simulink model "CACC_3_vehicles"  (R2021a)
settings: Solver=VariableStepAuto  StartTime=0.0  StopTime=120  RelTol=1e-3
values from neighbouring files (symbols this model uses):
  h = 0.9    [CACC_6_vehicles.m]    (also in CACC_6_vehicles_with_independent_FF_of_LeadVeh_Acceltn_Pstn.m; CACC_init.m)
  Kd = 1.2    [CACC_6_vehicles.m]    (also in CACC_6_vehicles_with_independent_FF_of_LeadVeh_Acceltn_Pstn.m; CACC_init.m)
  Kp = 1.5    [CACC_6_vehicles.m]    (also in CACC_6_vehicles_with_independent_FF_of_LeadVeh_Acceltn_Pstn.m; CACC_init.m)
  Lambda0 = 1    [CACC_6_vehicles.m]    (also in CACC_6_vehicles_with_independent_FF_of_LeadVeh_Acceltn_Pstn.m; CACC_init.m)
  Lambda1 = 0.5    [CACC_6_vehicles.m]    (also in CACC_6_vehicles_with_independent_FF_of_LeadVeh_Acceltn_Pstn.m; CACC_init.m)
  Lambda2 = 0.7    [CACC_6_vehicles.m]    (also in CACC_6_vehicles_with_independent_FF_of_LeadVeh_Acceltn_Pstn.m; CACC_init.m)
  Lambda3 = 0.75    [CACC_6_vehicles.m]    (also in CACC_6_vehicles_with_independent_FF_of_LeadVeh_Acceltn_Pstn.m; CACC_init.m)
  tau = 0.002    [CACC_6_vehicles.m]    (also in CACC_6_vehicles_with_independent_FF_of_LeadVeh_Acceltn_Pstn.m; CACC_init.m)
  tau0 = 0.1    [CACC_6_vehicles.m]    (also in CACC_6_vehicles_with_independent_FF_of_LeadVeh_Acceltn_Pstn.m; CACC_init.m)
  tau1 = 0.5    [CACC_6_vehicles.m]    (also in CACC_6_vehicles_with_independent_FF_of_LeadVeh_Acceltn_Pstn.m; CACC_init.m)
  tau2 = 0.7    [CACC_6_vehicles.m]    (also in CACC_6_vehicles_with_independent_FF_of_LeadVeh_Acceltn_Pstn.m; CACC_init.m)
  tau3 = 0.3    [CACC_6_vehicles.m]    (also in CACC_6_vehicles_with_independent_FF_of_LeadVeh_Acceltn_Pstn.m; CACC_init.m)
undefined symbols (not defined in the file or in its folder): sigbuilder_block
libraries: pid_lib x3
settings Model: Creator=ChOm1  LastModifiedBy=User
settings SolverCC: AlgebraicLoopSolver=TrustRegion
settings DebuggingCC: SFMachineParentedDataDiag=warning

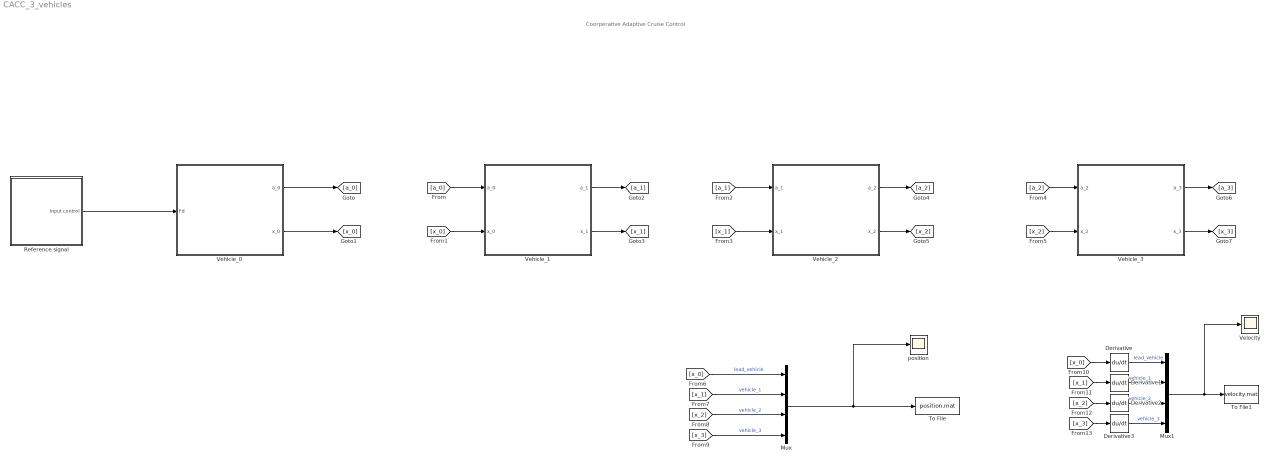
== system CACC_3_vehicles ==
  note: Coorperative Adaptive Cruise Control
  Derivative{,1..3} (4 alike) : Derivative
  Mux : Mux
  Mux1 : Mux
  Reference signal : Subsystem  Tag=STV Subsys  LoadFcn=sigbuilder_block('load');  StartFcn=sigbuilder_block('start');  StopFcn=sigbuilder_block('stop');  ClipboardFcn=sigbuilder_block('clipboard');  mask(Sigbuilder block){tuvar=[0:10]}
      mask help: Simulink:masks:SigbuilderBlock_MD
      mask init:
      | if ~strcmp(get_param(bdroot(gcbh),'SimulationStatus'),'stopped') tuvar = sigbuilder_block('maskInit'); end
      settings: CopyFcn=sigbuilder_block('copy');  DeleteFcn=sigbuilder_block('delete');  ModelCloseFcn=sigbuilder_block('modelClose');  PreSaveFcn=sigbuilder_block('preSave');  PauseFcn=sigbuilder_block('pause');  ContinueFcn=sigbuilder_block('continue');  NameChangeFcn=sigbuilder_block('namechange');  OpenFcn=sigbuilder_block('open',[259.5 231.75 543.75 273.75 ]);  CloseFcn=sigbuilder_block('close');
      mask Display: plot(0, 0, 100, 100,[2, 2, 32, 32, 2], [68, 8, 8, 68, 68],[32, 2], [38, 38], [32, 19, 2],[53, 60, 44], [32, 17, 17, 2],[16, 16, 31, 31]);txt = getActiveGroup(gcbh);text(2, 100, txt,'verticalAlignment', 'top');
  To File : ToFile  Filename=position.mat
  To File1 : ToFile  Filename=velocity.mat
  Vehicle_0 : Subsystem
  Vehicle_1 : Subsystem
  Vehicle_2 : Subsystem
  Vehicle_3 : Subsystem
  Velocity : Scope
  position : Scope
  wires:
  Reference signal/1(Input control) -> Vehicle_0/1(Fd)
  Vehicle_0/1(a_0) -> [a_0]
  Vehicle_0/2(x_0) -> [x_0]
  [a_0] -> Vehicle_1/1(a_0)
  [x_0] -> Vehicle_1/2(x_0)
  Vehicle_1/1(a_1) -> [a_1]
  [a_1] -> Vehicle_2/1(a_1)
  [x_1] -> Vehicle_2/2(x_1)
  Vehicle_2/1(a_2) -> [a_2]
  Vehicle_2/2(x_2) -> [x_2]
  [x_2] -> Vehicle_3/2(x_2)
  [a_2] -> Vehicle_3/1(a_2)
  Vehicle_3/1(a_3) -> [a_3]
  Vehicle_3/2(x_3) -> [x_3]
  Vehicle_1/2(x_1) -> [x_1]
  [x_0] -> Mux/1  "lead_vehicle"
  [x_1] -> Mux/2  "vehicle_1"
  [x_2] -> Mux/3  "vehicle_2"
  [x_3] -> Mux/4  "vehicle_3"
  Mux/1 -> position/1, To File/1
  [x_2] -> Derivative2/1
  Mux1/1 -> Velocity/1, To File1/1
  [x_0] -> Derivative/1
  Derivative/1 -> Mux1/1  "lead_vehicle"
  [x_1] -> Derivative1/1
  Derivative1/1 -> Mux1/2  "vehicle_1"
  Derivative2/1 -> Mux1/3  "vehicle_2"
  [x_3] -> Derivative3/1
  Derivative3/1 -> Mux1/4  "vehicle_3"

== system CACC_3_vehicles/Reference signal ==
  Demux : Demux  Tag=STV Demux  Outputs=1
      settings: DisplayOption=none
  FromWs : FromWorkspace  Tag=STV FromWs  VariableName=tuvar
      SigBuilderData=|
      | common.afterFinalStr = 'Extrapolate'
      | common.sampleTime = 0
      | dataSet.timeRange = [0 120]
      | dataSet.name = 'Group 1'
      | sbobj.Groups.Name = 'Group 1'
      | sbobj.Groups.Signals.Name = 'Input control'
      | sbobj.Groups.Signals.XData = [0 20.1 20.1 23.5 23.5 27.9 27.9 51.7 60.1 85.2 110.5 120]
      | sbobj.Groups.Signals.YData = [0 1.045 -1.5 -0.64 1.86 2.08 2.09 0 0 -2 0 0]
      | sbobj.Groups.TimeRange = [0 120]
  Input control : Outport  Tag=STV Outport
  wires:
  FromWs/1 -> Demux/1
  Demux/1 -> Input control/1

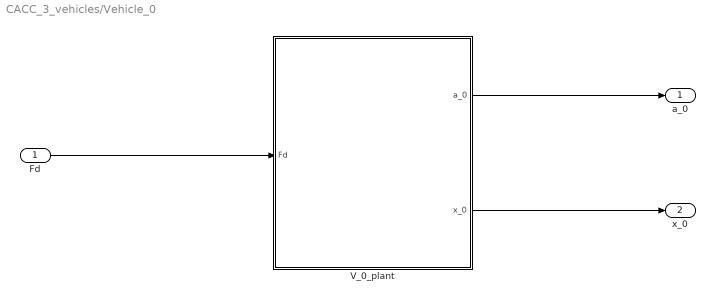
== system CACC_3_vehicles/Vehicle_0 ==
  Fd : Inport
  V_0_plant : Subsystem
  a_0 : Outport
  x_0 : Outport  Port=2
  wires:
  Fd/1 -> V_0_plant/1(Fd)
  V_0_plant/1(a_0) -> a_0/1
  V_0_plant/2(x_0) -> x_0/1

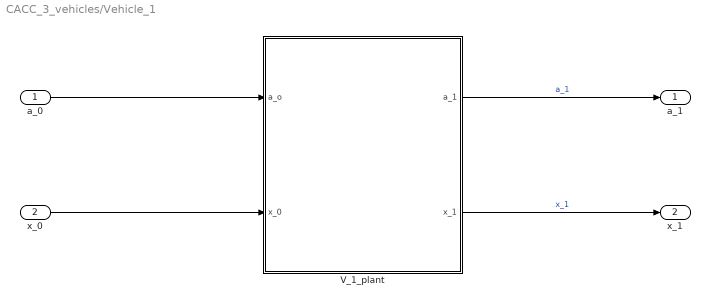
== system CACC_3_vehicles/Vehicle_1 ==
  a_0 : Inport
  x_0 : Inport  Port=2
  V_1_plant : Subsystem
  a_1 : Outport
  x_1 : Outport  Port=2
  wires:
  a_0/1 -> V_1_plant/1(a_o)
  x_0/1 -> V_1_plant/2(x_0)
  V_1_plant/1(a_1) -> a_1/1  "a_1"
  V_1_plant/2(x_1) -> x_1/1  "x_1"

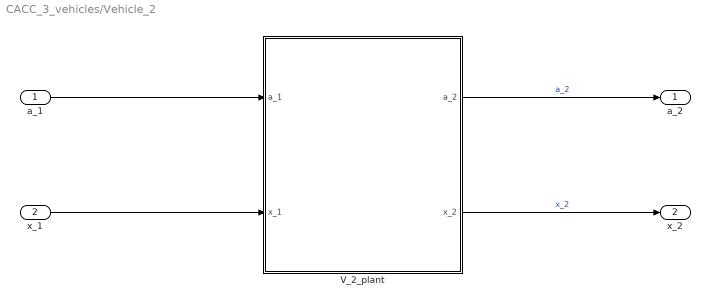
== system CACC_3_vehicles/Vehicle_2 ==
  a_1 : Inport
  x_1 : Inport  Port=2
  V_2_plant : Subsystem
  a_2 : Outport
  x_2 : Outport  Port=2
  wires:
  V_2_plant/2(x_2) -> x_2/1  "x_2"
  V_2_plant/1(a_2) -> a_2/1  "a_2"
  x_1/1 -> V_2_plant/2(x_1)
  a_1/1 -> V_2_plant/1(a_1)

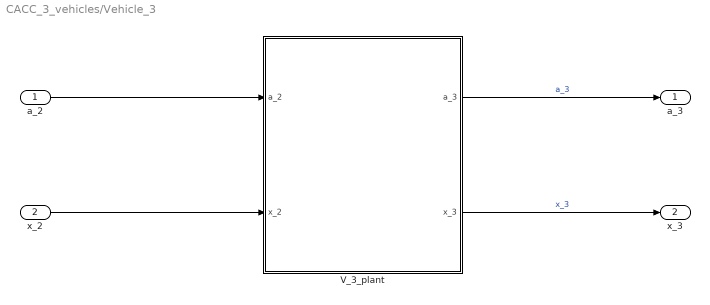
== system CACC_3_vehicles/Vehicle_3 ==
  a_2 : Inport
  x_2 : Inport  Port=2
  V_3_plant : Subsystem
  a_3 : Outport
  x_3 : Outport  Port=2
  wires:
  a_2/1 -> V_3_plant/1(a_2)
  x_2/1 -> V_3_plant/2(x_2)
  V_3_plant/1(a_3) -> a_3/1  "a_3"
  V_3_plant/2(x_3) -> x_3/1  "x_3"

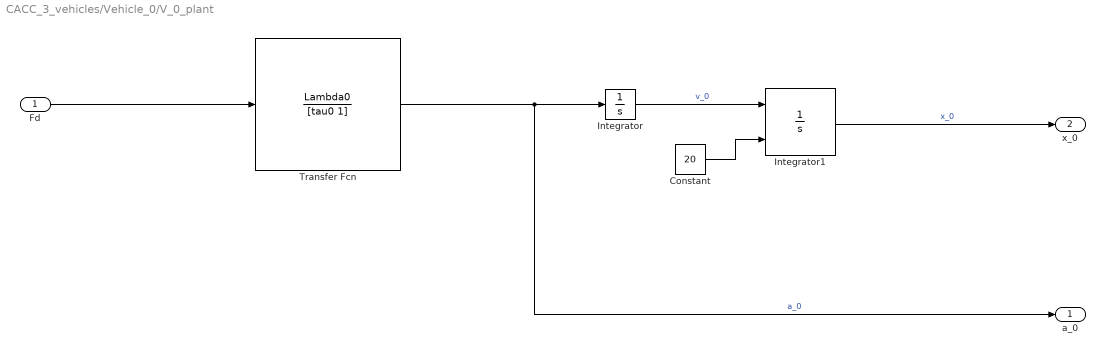
== system CACC_3_vehicles/Vehicle_0/V_0_plant ==
  Fd : Inport
  Constant : Constant  Value=20
  Integrator : Integrator
  Integrator1 : Integrator  InitialConditionSource=external
  Transfer Fcn : TransferFcn  Numerator=Lambda0  Denominator=[tau0 1]
  a_0 : Outport
  x_0 : Outport  Port=2
  wires:
  Fd/1 -> Transfer Fcn/1
  Transfer Fcn/1 -> a_0/1, Integrator/1  "a_0"
  Integrator/1 -> Integrator1/1  "v_0"
  Integrator1/1 -> x_0/1  "x_0"
  Constant/1 -> Integrator1/2

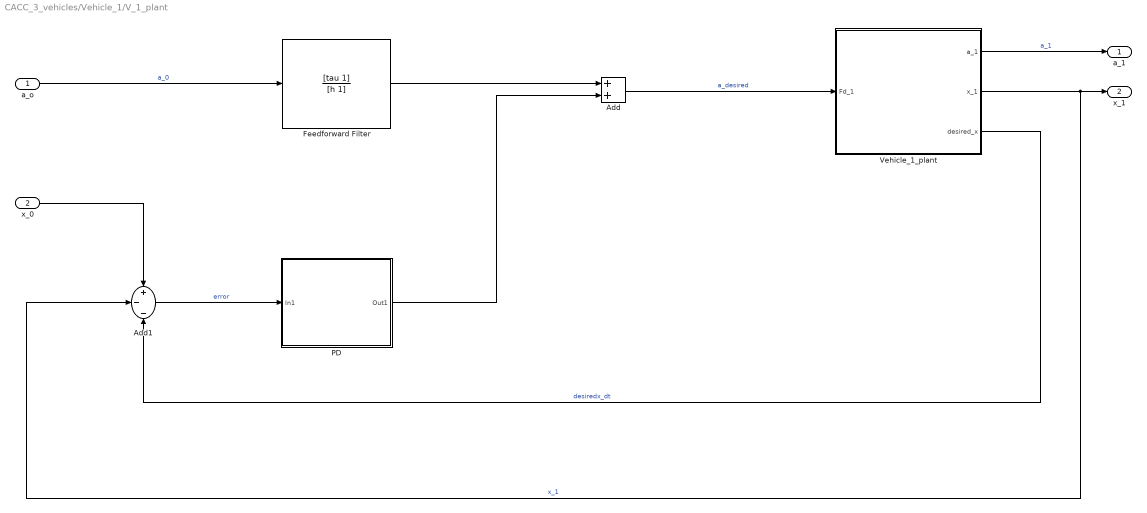
== system CACC_3_vehicles/Vehicle_1/V_1_plant ==
  a_o : Inport
  x_0 : Inport  Port=2
  Add : Sum
  Add1 : Sum  Inputs=+--
  Feedforward Filter : TransferFcn  Numerator=[tau 1]  Denominator=[h 1]
  PD : Subsystem
  Vehicle_1_plant : Subsystem
  a_1 : Outport
  x_1 : Outport  Port=2
  wires:
  a_o/1 -> Feedforward Filter/1  "a_0"
  Feedforward Filter/1 -> Add/1
  Add1/1 -> PD/1(In1)  "error"
  x_0/1 -> Add1/1
  PD/1(Out1) -> Add/2
  Add/1 -> Vehicle_1_plant/1(Fd_1)  "a_desired"
  Vehicle_1_plant/1(a_1) -> a_1/1  "a_1"
  Vehicle_1_plant/2(x_1) -> Add1/2, x_1/1  "x_1"
  Vehicle_1_plant/3(desired_x) -> Add1/3  "desiredx_dt"

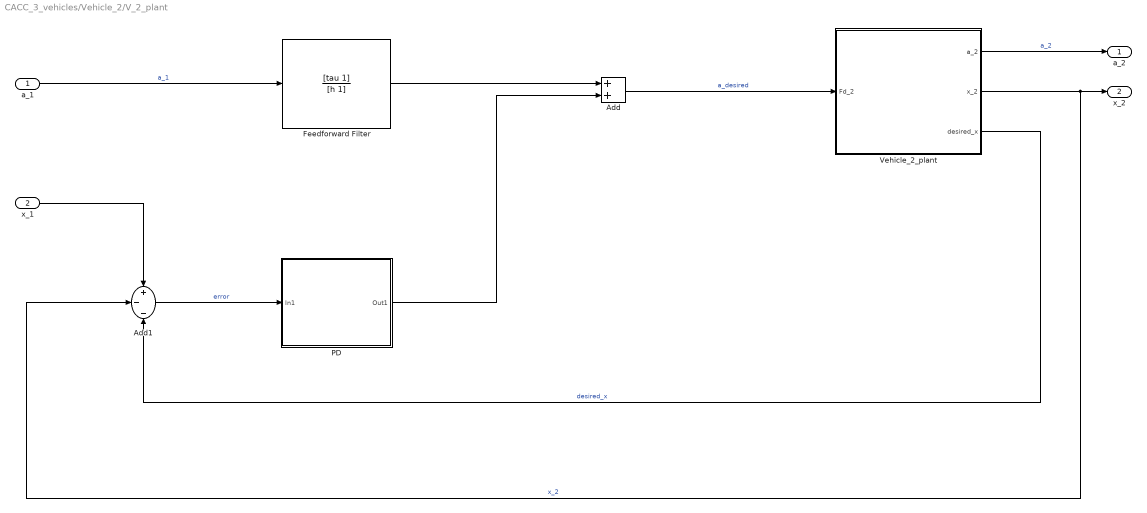
== system CACC_3_vehicles/Vehicle_2/V_2_plant ==
  a_1 : Inport
  x_1 : Inport  Port=2
  Add : Sum
  Add1 : Sum  Inputs=+--
  Feedforward Filter : TransferFcn  Numerator=[tau 1]  Denominator=[h 1]
  PD : Subsystem
  Vehicle_2_plant : Subsystem
  a_2 : Outport
  x_2 : Outport  Port=2
  wires:
  Vehicle_2_plant/3(desired_x) -> Add1/3  "desired_x"
  Vehicle_2_plant/2(x_2) -> x_2/1, Add1/2  "x_2"
  Vehicle_2_plant/1(a_2) -> a_2/1  "a_2"
  Add/1 -> Vehicle_2_plant/1(Fd_2)  "a_desired"
  PD/1(Out1) -> Add/2
  x_1/1 -> Add1/1
  Add1/1 -> PD/1(In1)  "error"
  Feedforward Filter/1 -> Add/1
  a_1/1 -> Feedforward Filter/1  "a_1"

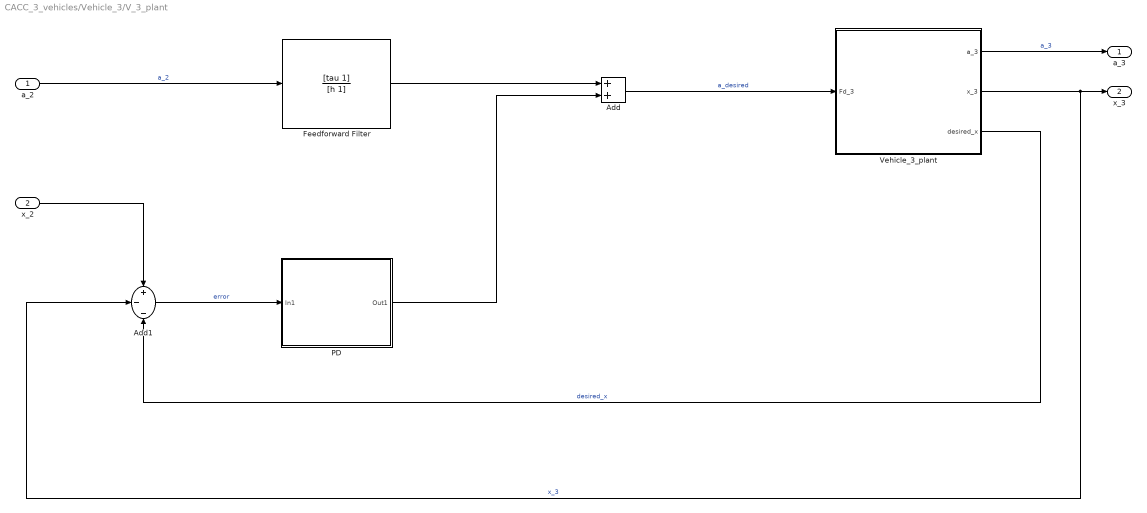
== system CACC_3_vehicles/Vehicle_3/V_3_plant ==
  a_2 : Inport
  x_2 : Inport  Port=2
  Add : Sum
  Add1 : Sum  Inputs=+--
  Feedforward Filter : TransferFcn  Numerator=[tau 1]  Denominator=[h 1]
  PD : Subsystem
  Vehicle_3_plant : Subsystem
  a_3 : Outport
  x_3 : Outport  Port=2
  wires:
  a_2/1 -> Feedforward Filter/1  "a_2"
  Feedforward Filter/1 -> Add/1
  Add1/1 -> PD/1(In1)  "error"
  x_2/1 -> Add1/1
  PD/1(Out1) -> Add/2
  Add/1 -> Vehicle_3_plant/1(Fd_3)  "a_desired"
  Vehicle_3_plant/1(a_3) -> a_3/1  "a_3"
  Vehicle_3_plant/2(x_3) -> Add1/2, x_3/1  "x_3"
  Vehicle_3_plant/3(desired_x) -> Add1/3  "desired_x"

== system CACC_3_vehicles/Vehicle_1/V_1_plant/PD ==
  In1 : Inport
  PID Controller : pid_lib/PID Controller  Controller=PID  Form=Parallel  TimeDomain=Continuous-time  UseExternalTs=off  SampleTime=-1  IntegratorMethod=Forward Euler  FilterMethod=Forward Euler  ControllerParametersSource=internal  P=Kp  I=0  D=Kd  UseFilter=on  N=100  TunerSelectOption=Transfer Function Based (PID Tuner App)  InitialConditionSource=internal  InitialConditionForIntegrator=0  InitialConditionForFilter=0  DifferentiatorICPrevScaledInput=0  ExternalReset=none  TrackingMode=off  Kt=1  LimitOutput=off  SatLimitsSource=internal  UpperSaturationLimit=inf  LowerSaturationLimit=-inf  LinearizeAsGain=on  AntiWindupMode=none  Kb=1  POutMin=[]  POutMax=[]  IOutMin=[]  IOutMax=[]  DOutMin=[]  DOutMax=[]  NOutMin=[]  NOutMax=[]  SumOutMin=[]  SumOutMax=[]  SaturationOutMin=[]  SaturationOutMax=[]  PParamMin=[]  PParamMax=[]  IParamMin=[]  IParamMax=[]  DParamMin=[]  DParamMax=[]  NParamMin=[]  NParamMax=[]  KbParamMin=[]  KbParamMax=[]  KtParamMin=[]  KtParamMax=[]  KbOutMin=[]  KbOutMax=[]  KtOutMin=[]  KtOutMax=[]  IntegratorOutMin=[]  IntegratorOutMax=[]  FilterOutMin=[]  FilterOutMax=[]  SumI1OutMin=[]  SumI1OutMax=[]  SumI2OutMin=[]  SumI2OutMax=[]  SumI3OutMin=[]  SumI3OutMax=[]  SumI4OutMin=[]  SumI4OutMax=[]  SumDOutMin=[]  SumDOutMax=[]  DifferentiatorOutMin=[]  DifferentiatorOutMax=[]  FilterDiffOutCoefMin=[]  FilterDiffOutCoefMax=[]  ReciprocalOutMin=[]  ReciprocalOutMax=[]  SumDenOutMin=[]  SumDenOutMax=[]  SumNumOutMin=[]  SumNumOutMax=[]  DivideOutMin=[]  DivideOutMax=[]  UdiffTsProdOutMin=[]  UdiffTsProdOutMax=[]  NTsProdOutMin=[]  NTsProdOutMax=[]  UintegralTsProdOutMin=[]  UintegralTsProdOutMax=[]  UngainTsProdOutMin=[]  UngainTsProdOutMax=[]  IntegratorContinuousStateAttributes=''  IntegratorStateMustResolveToSignalObject=off  IntegratorRTWStateStorageClass=Auto  FilterContinuousStateAttributes=''  FilterStateMustResolveToSignalObject=off  FilterRTWStateStorageClass=Auto  ParallelPVariant=InternalParameters  IdealPVariant=Disabled  IVariant=InternalParameters  DVariant=InternalParameters  IntegratorVariant=Continuous  SatVariant=Disabled  AWVariant=Passthrough  PCopyVariant=Disabled  TRVariant=Disabled  FdbkBlocksVariant=Forward  IdealPFdbkVariant=Disabled  SatFdbkVariant=Disabled  DerivativeFilterVariant=ContFilter  NVariant=InternalParameters  NCopyVariant=Disabled  FilterICVariant=InternalICsFilter  IntegratorICVariant=InternalICs  ExternalResetVariant=Disabled  TRSumVariant=Passthrough  SumFdbkVariant=Disabled  SumVariant=Sum_PID  TsampFilterVariant=InternalTs  TsampNgainVariant=Passthrough  TsampIntegralVariant=Passthrough  ExternalSaturationOutDataTypeStr=Inherit: Same as second input
  Out1 : Outport
  wires:
  In1/1 -> PID Controller/1
  PID Controller/1 -> Out1/1

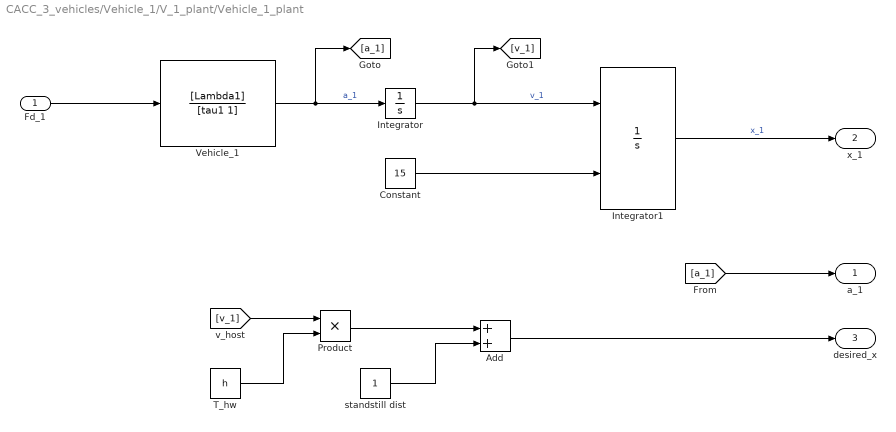
== system CACC_3_vehicles/Vehicle_1/V_1_plant/Vehicle_1_plant ==
  Fd_1 : Inport
  Add : Sum
  Constant : Constant  Value=15
  Integrator : Integrator
  Integrator1 : Integrator  InitialConditionSource=external
  Product : Product
  T_hw : Constant  Value=h
  Vehicle_1 : TransferFcn  Numerator=[Lambda1]  Denominator=[tau1 1]
  standstill dist : Constant
  a_1 : Outport
  x_1 : Outport  Port=2
  desired_x : Outport  Port=3
  wires:
  Fd_1/1 -> Vehicle_1/1
  Vehicle_1/1 -> [a_1], Integrator/1  "a_1"
  Integrator/1 -> [v_1], Integrator1/1  "v_1"
  Integrator1/1 -> x_1/1  "x_1"
  Constant/1 -> Integrator1/2
  [a_1] -> a_1/1
  [v_1] -> Product/1
  T_hw/1 -> Product/2
  Product/1 -> Add/1
  Add/1 -> desired_x/1
  standstill dist/1 -> Add/2

== system CACC_3_vehicles/Vehicle_2/V_2_plant/PD ==
  In1 : Inport
  PID Controller : pid_lib/PID Controller  Controller=PID  Form=Parallel  TimeDomain=Continuous-time  UseExternalTs=off  SampleTime=-1  IntegratorMethod=Forward Euler  FilterMethod=Forward Euler  ControllerParametersSource=internal  P=Kp  I=0  D=Kd  UseFilter=on  N=100  TunerSelectOption=Transfer Function Based (PID Tuner App)  InitialConditionSource=internal  InitialConditionForIntegrator=0  InitialConditionForFilter=0  DifferentiatorICPrevScaledInput=0  ExternalReset=none  TrackingMode=off  Kt=1  LimitOutput=off  SatLimitsSource=internal  UpperSaturationLimit=inf  LowerSaturationLimit=-inf  LinearizeAsGain=on  AntiWindupMode=none  Kb=1  POutMin=[]  POutMax=[]  IOutMin=[]  IOutMax=[]  DOutMin=[]  DOutMax=[]  NOutMin=[]  NOutMax=[]  SumOutMin=[]  SumOutMax=[]  SaturationOutMin=[]  SaturationOutMax=[]  PParamMin=[]  PParamMax=[]  IParamMin=[]  IParamMax=[]  DParamMin=[]  DParamMax=[]  NParamMin=[]  NParamMax=[]  KbParamMin=[]  KbParamMax=[]  KtParamMin=[]  KtParamMax=[]  KbOutMin=[]  KbOutMax=[]  KtOutMin=[]  KtOutMax=[]  IntegratorOutMin=[]  IntegratorOutMax=[]  FilterOutMin=[]  FilterOutMax=[]  SumI1OutMin=[]  SumI1OutMax=[]  SumI2OutMin=[]  SumI2OutMax=[]  SumI3OutMin=[]  SumI3OutMax=[]  SumI4OutMin=[]  SumI4OutMax=[]  SumDOutMin=[]  SumDOutMax=[]  DifferentiatorOutMin=[]  DifferentiatorOutMax=[]  FilterDiffOutCoefMin=[]  FilterDiffOutCoefMax=[]  ReciprocalOutMin=[]  ReciprocalOutMax=[]  SumDenOutMin=[]  SumDenOutMax=[]  SumNumOutMin=[]  SumNumOutMax=[]  DivideOutMin=[]  DivideOutMax=[]  UdiffTsProdOutMin=[]  UdiffTsProdOutMax=[]  NTsProdOutMin=[]  NTsProdOutMax=[]  UintegralTsProdOutMin=[]  UintegralTsProdOutMax=[]  UngainTsProdOutMin=[]  UngainTsProdOutMax=[]  IntegratorContinuousStateAttributes=''  IntegratorStateMustResolveToSignalObject=off  IntegratorRTWStateStorageClass=Auto  FilterContinuousStateAttributes=''  FilterStateMustResolveToSignalObject=off  FilterRTWStateStorageClass=Auto  ParallelPVariant=InternalParameters  IdealPVariant=Disabled  IVariant=InternalParameters  DVariant=InternalParameters  IntegratorVariant=Continuous  SatVariant=Disabled  AWVariant=Passthrough  PCopyVariant=Disabled  TRVariant=Disabled  FdbkBlocksVariant=Forward  IdealPFdbkVariant=Disabled  SatFdbkVariant=Disabled  DerivativeFilterVariant=ContFilter  NVariant=InternalParameters  NCopyVariant=Disabled  FilterICVariant=InternalICsFilter  IntegratorICVariant=InternalICs  ExternalResetVariant=Disabled  TRSumVariant=Passthrough  SumFdbkVariant=Disabled  SumVariant=Sum_PID  TsampFilterVariant=InternalTs  TsampNgainVariant=Passthrough  TsampIntegralVariant=Passthrough  ExternalSaturationOutDataTypeStr=Inherit: Same as second input
  Out1 : Outport
  wires:
  PID Controller/1 -> Out1/1
  In1/1 -> PID Controller/1

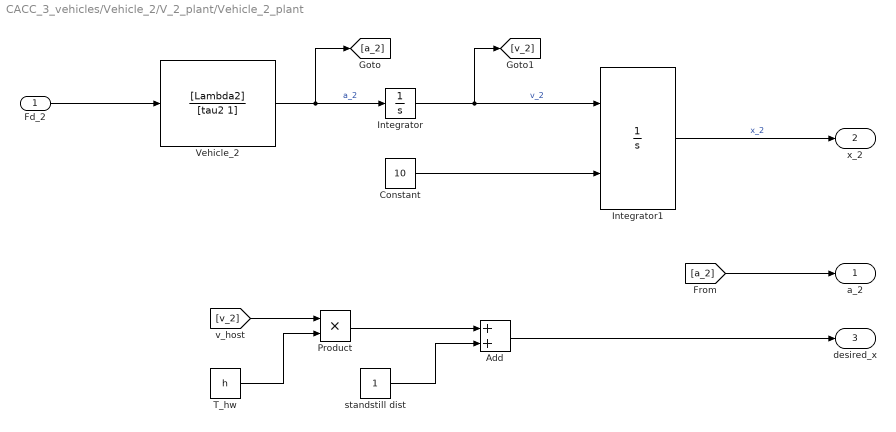
== system CACC_3_vehicles/Vehicle_2/V_2_plant/Vehicle_2_plant ==
  Fd_2 : Inport
  Add : Sum
  Constant : Constant  Value=10
  Integrator : Integrator
  Integrator1 : Integrator  InitialConditionSource=external
  Product : Product
  T_hw : Constant  Value=h
  Vehicle_2 : TransferFcn  Numerator=[Lambda2]  Denominator=[tau2 1]
  standstill dist : Constant
  a_2 : Outport
  x_2 : Outport  Port=2
  desired_x : Outport  Port=3
  wires:
  Add/1 -> desired_x/1
  Product/1 -> Add/1
  T_hw/1 -> Product/2
  [v_2] -> Product/1
  [a_2] -> a_2/1
  Constant/1 -> Integrator1/2
  Integrator1/1 -> x_2/1  "x_2"
  Integrator/1 -> Integrator1/1, [v_2]  "v_2"
  Vehicle_2/1 -> Integrator/1, [a_2]  "a_2"
  Fd_2/1 -> Vehicle_2/1
  standstill dist/1 -> Add/2

== system CACC_3_vehicles/Vehicle_3/V_3_plant/PD ==
  In1 : Inport
  PID Controller : pid_lib/PID Controller  Controller=PID  Form=Parallel  TimeDomain=Continuous-time  UseExternalTs=off  SampleTime=-1  IntegratorMethod=Forward Euler  FilterMethod=Forward Euler  ControllerParametersSource=internal  P=Kp  I=0  D=Kd  UseFilter=on  N=100  TunerSelectOption=Transfer Function Based (PID Tuner App)  InitialConditionSource=internal  InitialConditionForIntegrator=0  InitialConditionForFilter=0  DifferentiatorICPrevScaledInput=0  ExternalReset=none  TrackingMode=off  Kt=1  LimitOutput=off  SatLimitsSource=internal  UpperSaturationLimit=inf  LowerSaturationLimit=-inf  LinearizeAsGain=on  AntiWindupMode=none  Kb=1  POutMin=[]  POutMax=[]  IOutMin=[]  IOutMax=[]  DOutMin=[]  DOutMax=[]  NOutMin=[]  NOutMax=[]  SumOutMin=[]  SumOutMax=[]  SaturationOutMin=[]  SaturationOutMax=[]  PParamMin=[]  PParamMax=[]  IParamMin=[]  IParamMax=[]  DParamMin=[]  DParamMax=[]  NParamMin=[]  NParamMax=[]  KbParamMin=[]  KbParamMax=[]  KtParamMin=[]  KtParamMax=[]  KbOutMin=[]  KbOutMax=[]  KtOutMin=[]  KtOutMax=[]  IntegratorOutMin=[]  IntegratorOutMax=[]  FilterOutMin=[]  FilterOutMax=[]  SumI1OutMin=[]  SumI1OutMax=[]  SumI2OutMin=[]  SumI2OutMax=[]  SumI3OutMin=[]  SumI3OutMax=[]  SumI4OutMin=[]  SumI4OutMax=[]  SumDOutMin=[]  SumDOutMax=[]  DifferentiatorOutMin=[]  DifferentiatorOutMax=[]  FilterDiffOutCoefMin=[]  FilterDiffOutCoefMax=[]  ReciprocalOutMin=[]  ReciprocalOutMax=[]  SumDenOutMin=[]  SumDenOutMax=[]  SumNumOutMin=[]  SumNumOutMax=[]  DivideOutMin=[]  DivideOutMax=[]  UdiffTsProdOutMin=[]  UdiffTsProdOutMax=[]  NTsProdOutMin=[]  NTsProdOutMax=[]  UintegralTsProdOutMin=[]  UintegralTsProdOutMax=[]  UngainTsProdOutMin=[]  UngainTsProdOutMax=[]  IntegratorContinuousStateAttributes=''  IntegratorStateMustResolveToSignalObject=off  IntegratorRTWStateStorageClass=Auto  FilterContinuousStateAttributes=''  FilterStateMustResolveToSignalObject=off  FilterRTWStateStorageClass=Auto  ParallelPVariant=InternalParameters  IdealPVariant=Disabled  IVariant=InternalParameters  DVariant=InternalParameters  IntegratorVariant=Continuous  SatVariant=Disabled  AWVariant=Passthrough  PCopyVariant=Disabled  TRVariant=Disabled  FdbkBlocksVariant=Forward  IdealPFdbkVariant=Disabled  SatFdbkVariant=Disabled  DerivativeFilterVariant=ContFilter  NVariant=InternalParameters  NCopyVariant=Disabled  FilterICVariant=InternalICsFilter  IntegratorICVariant=InternalICs  ExternalResetVariant=Disabled  TRSumVariant=Passthrough  SumFdbkVariant=Disabled  SumVariant=Sum_PID  TsampFilterVariant=InternalTs  TsampNgainVariant=Passthrough  TsampIntegralVariant=Passthrough  ExternalSaturationOutDataTypeStr=Inherit: Same as second input
  Out1 : Outport
  wires:
  In1/1 -> PID Controller/1
  PID Controller/1 -> Out1/1

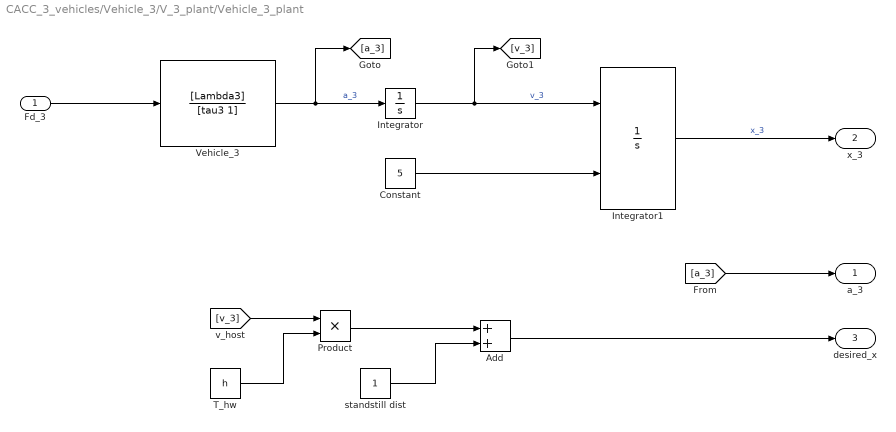
== system CACC_3_vehicles/Vehicle_3/V_3_plant/Vehicle_3_plant ==
  Fd_3 : Inport
  Add : Sum
  Constant : Constant  Value=5
  Integrator : Integrator
  Integrator1 : Integrator  InitialConditionSource=external
  Product : Product
  T_hw : Constant  Value=h
  Vehicle_3 : TransferFcn  Numerator=[Lambda3]  Denominator=[tau3 1]
  standstill dist : Constant
  a_3 : Outport
  x_3 : Outport  Port=2
  desired_x : Outport  Port=3
  wires:
  standstill dist/1 -> Add/2
  Fd_3/1 -> Vehicle_3/1
  Vehicle_3/1 -> [a_3], Integrator/1  "a_3"
  Integrator/1 -> [v_3], Integrator1/1  "v_3"
  Integrator1/1 -> x_3/1  "x_3"
  Constant/1 -> Integrator1/2
  [a_3] -> a_3/1
  [v_3] -> Product/1
  T_hw/1 -> Product/2
  Product/1 -> Add/1
  Add/1 -> desired_x/1
